simulink model "ctrl_1khz"  (R2017a)
settings: Solver=FixedStepAuto  StartTime=0.0  StopTime=10.0  FixedStep=1e-3  RelTol=1e-3  EnableMultiTasking=on
undefined symbols (not defined in the file): Spd_PI_Ki, Spd_PI_Kp
settings Model: Creator=uids8840  LastModifiedBy=root
settings SolverCC: AutoInsertRateTranBlk=on
settings DataIOCC: SaveOutput=off  SignalLogging=off  DSMLogging=off  SaveTime=off
settings OptimizationCC: DefaultParameterBehavior=Inlined  UseFloatMulNetSlope=on  DefaultUnderspecifiedDataType=single  InlineInvariantSignals=on  PassReuseOutputArgsAs=Individual arguments  ZeroExternalMemoryAtStartup=off  ZeroInternalMemoryAtStartup=off  NoFixptDivByZeroProtection=on  EfficientFloat2IntCast=on  LifeSpan=1
settings DebuggingCC: ParameterTunabilityLossMsg=error
settings HardwareCC: ProdBitPerPointer=32  ProdBitPerSizeT=32  ProdBitPerPtrDiffT=32  ProdLargestAtomicInteger=Long  ProdWordSize=32  ProdHWDeviceType=ARM Compatible->ARM 10  TargetBitPerLong=64  TargetBitPerPointer=64  TargetBitPerSizeT=64  TargetBitPerPtrDiffT=64  TargetLongLongMode=on  TargetIntDivRoundTo=Zero  TargetEndianess=LittleEndian  TargetWordSize=64  TargetHWDeviceType=Generic->MATLAB Host Computer
settings ModelReferenceCC: ModelReferenceNumInstancesAllowed=Single
settings SFSimCC: MATLABDynamicMemAlloc=off
settings RTWCC: SystemTargetFile=ert.tlc  GenCodeOnly=on  PackageGeneratedCodeAndArtifacts=on  PackageName=mtrctl  TemplateMakefile=ert_default_tmf  Description=Embedded Coder  GenerateReport=on  IncludeHyperlinkInReport=on  LaunchReport=on  PortableWordSizes=on  GenerateTraceInfo=on  GenerateTraceReport=on  GenerateTraceReportSl=on  GenerateTraceReportSf=on  GenerateTraceReportEml=on  GenerateCodeMetricsReport=on
settings CodeAppCC: ForceParamTrailComments=on  IgnoreCustomStorageClasses=off  OperatorAnnotations=on  SimulinkDataObjDesc=on  SFDataObjDesc=on  CustomSymbolStrGlobalVar=rt$N$M  CustomSymbolStrType=$N$M  CustomSymbolStrFcn=$N$M$F  CustomSymbolStrMacro=$N$M  InsertBlockDesc=on
settings ERTTargetCC: TargetLangStandard=C99 (ISO)  GenerateFullHeader=off  IncludeMdlTerminateFcn=off  CombineSignalStateStructs=on  SuppressErrorStatus=on  ERTCustomFileBanners=off  SupportAbsoluteTime=off  SupportNonFinite=off  SupportComplex=off  InlinedParameterPlacement=NonHierarchical  ERTCustomFileTemplate=example_file_process.tlc  GlobalDataDefinition=InSourceFile  GlobalDataReference=InSourceFile  ERTFilePackagingFormat=CompactWithDataFile

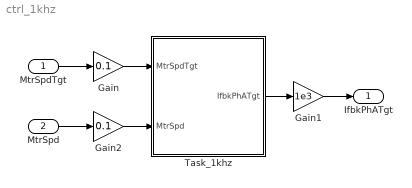
== system ctrl_1khz ==
  MtrSpdTgt : Inport
  MtrSpd : Inport  Port=2
  Gain : Gain  Gain=0.1
  Gain1 : Gain  Gain=1e3
  Gain2 : Gain  Gain=0.1
  Task_1khz : Subsystem  SystemSampleTime=1/1e3
  IfbkPhATgt : Outport
  wires:
  MtrSpdTgt/1 -> Gain/1
  MtrSpd/1 -> Gain2/1
  Gain/1 -> Task_1khz/1(MtrSpdTgt)
  Gain2/1 -> Task_1khz/2(MtrSpd)
  Task_1khz/1(IfbkPhATgt) -> Gain1/1
  Gain1/1 -> IfbkPhATgt/1

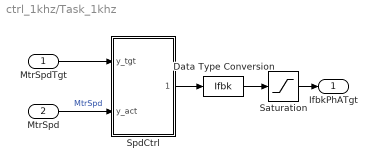
== system ctrl_1khz/Task_1khz ==
  MtrSpdTgt : Inport
  MtrSpd : Inport  Port=2
  Data Type Conversion : DataTypeConversion  OutDataTypeStr=Ifbk
  Saturation : Saturate  UpperLimit=2.  LowerLimit=-2.
  SpdCtrl : Subsystem  SystemSampleTime=ts  mask{ts=1e-3, PI_Kp=Spd_PI_Kp, PI_Ki=Spd_PI_Ki}
      mask prompts: ts "Execution Rate [s]:"; PI_Kp "Proportional Gain:"; PI_Ki "Integral Gain:"
      mask DialogControl DescTextVar Prompt: Discrete PI Controller.
  IfbkPhATgt : Outport
  wires:
  MtrSpd/1 -> SpdCtrl/2(y_act)  "MtrSpd"
  Data Type Conversion/1 -> Saturation/1
  SpdCtrl/1(PI_out) -> Data Type Conversion/1
  MtrSpdTgt/1 -> SpdCtrl/1(y_tgt)
  Saturation/1 -> IfbkPhATgt/1

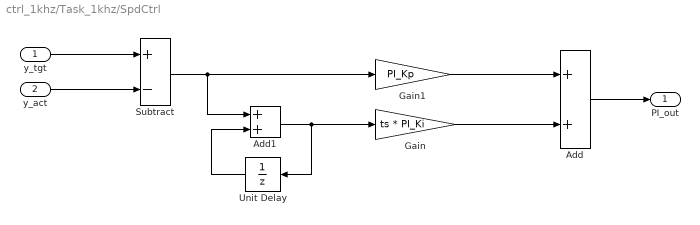
== system ctrl_1khz/Task_1khz/SpdCtrl ==
  y_tgt : Inport
  y_act : Inport  Port=2
  Add : Sum  OutDataTypeStr=Inherit: Inherit via back propagation
  Add1 : Sum
  Gain : Gain  Gain=ts * PI_Ki  ParamDataTypeStr=Inherit: Inherit from 'Gain'  OutDataTypeStr=Inherit: Inherit via back propagation
  Gain1 : Gain  Gain=PI_Kp  ParamDataTypeStr=Inherit: Inherit from 'Gain'  OutDataTypeStr=Inherit: Inherit via back propagation
  Subtract : Sum  Inputs=+-
  Unit Delay : UnitDelay  SampleTime=-1  StateName=ctrlstate
  PI_out : Outport
  wires:
  Add/1 -> PI_out/1
  y_act/1 -> Subtract/2
  Gain1/1 -> Add/1
  Subtract/1 -> Add1/1, Gain1/1
  y_tgt/1 -> Subtract/1
  Add1/1 -> Unit Delay/1, Gain/1
  Gain/1 -> Add/2
  Unit Delay/1 -> Add1/2
